simulink model "dev_lab6_XX"  (R2015b)
settings: Solver=ode3  StartTime=0.0  StopTime=2  FixedStep=2e-6  RelTol=1e-5
libraries: commfilt2 x1, commchan3 x1, commsink2 x1, commanapbnd3 x1, commrandsrc2 x1
settings Model: Creator=Dennis Silage  LastModifiedBy=trejo
settings DataIOCC: SaveFormat=Array  SignalLoggingSaveFormat=ModelDataLogs
settings OptimizationCC: ExpressionDepthLimit=2147483647  InitFltsAndDblsToZero=on
settings DebuggingCC: UnderspecifiedInitializationDetection=Classic  MergeDetectMultiDrivingBlocksExec=none  FcnCallInpInsideContextMsg=UseLocalSettings  StateNameClashWarn=warning
settings HardwareCC: ProdBitPerPointer=32  ProdLargestAtomicFloat=None  ProdIntDivRoundTo=Undefined  ProdEndianess=Unspecified  ProdWordSize=32  ProdHWDeviceType=32-bit Generic
settings GRTTargetCC: CombineOutputUpdateFcns=off  GRTInterface=on
settings ConfigComp: CovModelRefEnable=Off

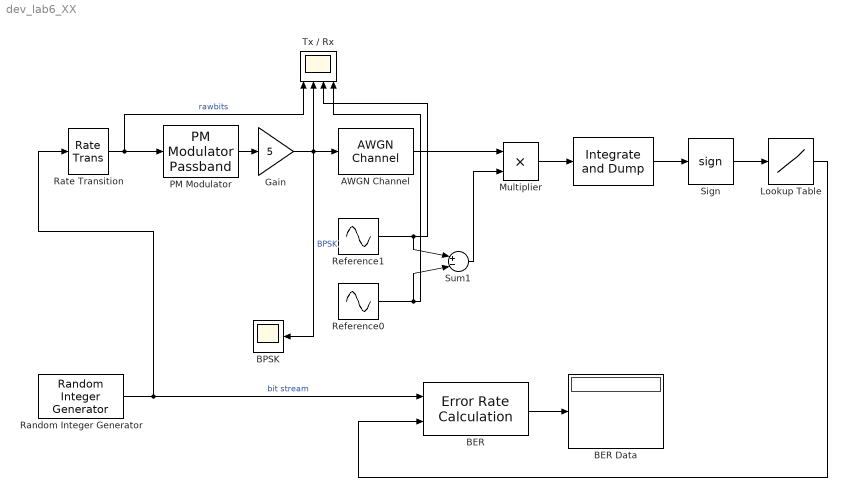
== system dev_lab6_XX ==
  " " : commfilt2/Integrate and Dump  obssamples=500  offsetsamples=0  nodump=off  roundingMode=Floor  overflowMode=off
  AWGN Channel : commchan3/AWGN Channel  InputProcessing=Inherited (this choice will be removed - see release notes)  seed=randseed  noiseMode="Signal to noise ratio  (Eb/No)"  EbNodB=50  EsNodB=10  SNRdB=12  bitsPerSym=1  Ps=12.5  Tsym=1e-3  variance=0
  BER : commsink2/Error Rate Calculation  N=2  st_delay=0  cp_mode=Entire frame  subframe=[]  PMode=Port  WsName=ErrorVec  RsMode2=off  stop=off  numErr=100  maxBits=1e6
  BER Data : Display
  BPSK : Scope
  Gain : Gain  Gain=5
  Lookup Table : Lookup  InputValues=[-1,0,1]  Table=[0,0,1]
  Multiplier : Product  RndMeth=Zero
  PM Modulator : commanapbnd3/PM Modulator Passband  Fc=20000  Ph=-25*pi/(180)  Kc=75*pi/(180)
  Random Integer Generator : commrandsrc2/Random Integer Generator  mul=2  seed=randseed  Ts=1e-3  frameBased=off  sampPerFrame=50  orient=on  outDataType=double
  Rate Transition : RateTransition  OutPortSampleTime=2e-6
  Reference0 : Sin  Amplitude=5  Frequency=20000*2*pi  Phase=-25*pi/180  Samples=200  SampleTime=2e-6
  Reference1 : Sin  Amplitude=5  Frequency=20000*2*pi  Phase=50*pi/180  Samples=200  SampleTime=2e-6
  Sign : Signum
  Sum1 : Sum  Inputs=|+-|
  Tx / Rx : Scope  NumInputPorts=4
  wires:
  Sign/1 -> Lookup Table/1
  BER/1 -> BER Data/1
  Multiplier/1 -> " "/1
  " "/1 -> Sign/1
  AWGN Channel/1 -> Multiplier/1
  Random Integer Generator/1 -> Rate Transition/1, BER/1  "bit stream"
  Gain/1 -> AWGN Channel/1, Tx / Rx/2, BPSK/1  "BPSK"
  Rate Transition/1 -> Tx / Rx/1, PM Modulator/1  "rawbits"
  PM Modulator/1 -> Gain/1
  Lookup Table/1 -> BER/2
  Reference1/1 -> Tx / Rx/3, Sum1/1
  Sum1/1 -> Multiplier/2
  Reference0/1 -> Tx / Rx/4, Sum1/2
